simulink model "cybershipII_ctrl_1_nonlin"  (R2020b)
settings: Solver=FixedStepAuto  StartTime=0.0  StopTime=100  FixedStep=0.01  RelTol=1e-3
libraries: simulink x1
settings Model: Creator=ASUS  LastModifiedBy=ASUS

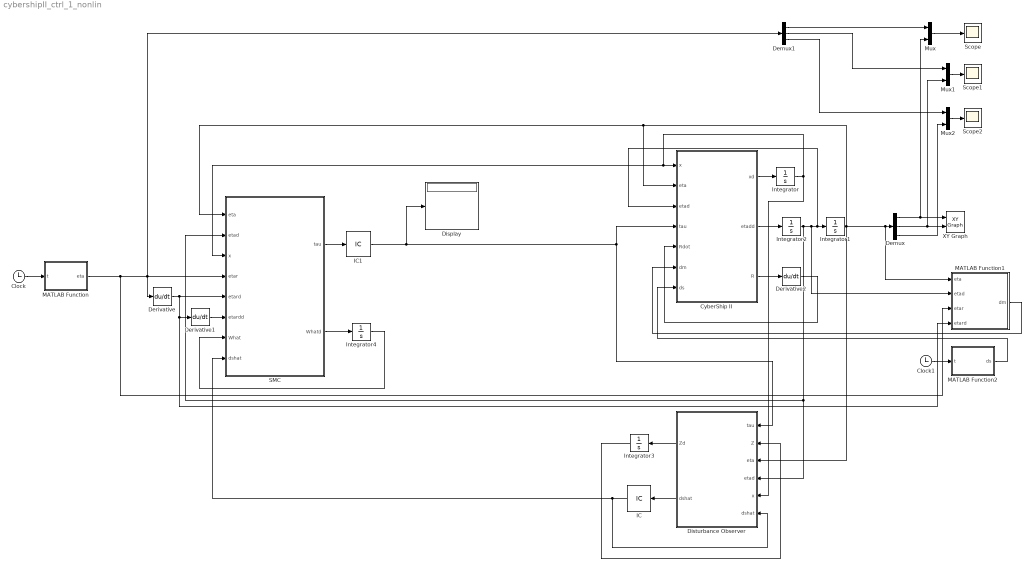
== system cybershipII_ctrl_1_nonlin ==
  Clock : Clock
  Clock1 : Clock
  CyberShip II : MATLAB Function  TreatAsAtomicUnit=on
  Demux : Demux  Outputs=3
  Demux1 : Demux  Outputs=3
  Derivative : Derivative
  Derivative1 : Derivative
  Derivative2 : Derivative
  Display : Display
  Disturbance Observer : MATLAB Function  TreatAsAtomicUnit=on
  IC : InitialCondition  Value=[0; 0; 0]
  IC1 : InitialCondition  Value=[0; 0; 0]
  Integrator : Integrator  InitialCondition=[3; 0; 0]
  Integrator1 : Integrator  InitialCondition=[0; 0; pi/4]
  Integrator2 : Integrator  InitialCondition=[3*cos(pi/4) 3*sin(pi/4) 0]
  Integrator3 : Integrator
  Integrator4 : Integrator
  MATLAB Function : MATLAB Function  TreatAsAtomicUnit=on
  MATLAB Function1 : MATLAB Function  TreatAsAtomicUnit=on
  MATLAB Function2 : MATLAB Function  TreatAsAtomicUnit=on
  Mux : Mux  Inputs=2
  Mux1 : Mux  Inputs=2
  Mux2 : Mux  Inputs=2
  SMC : MATLAB Function  TreatAsAtomicUnit=on
  Scope : Scope
  Scope1 : Scope
  Scope2 : Scope
  XY Graph : simulink/Sinks/XY Graph  xmin=-100  xmax=100  ymin=-100  ymax=100  st=-1
  wires:
  CyberShip II/1(xd) -> Integrator/1
  Integrator1/1 -> SMC/1(eta), CyberShip II/2(eta), MATLAB Function1/1(eta), Demux/1, Disturbance Observer/3(eta)
  Demux/1 -> Mux/2, XY Graph/1
  Demux/2 -> Mux1/2, XY Graph/2
  CyberShip II/3(R) -> Derivative2/1
  Derivative2/1 -> CyberShip II/5(Rdot)
  Integrator/1 -> Disturbance Observer/5(x), SMC/3(x), CyberShip II/1(x)
  CyberShip II/2(etadd) -> Integrator2/1
  Integrator2/1 -> SMC/2(etad), Disturbance Observer/4(etad), MATLAB Function1/2(etad), CyberShip II/3(etad), Integrator1/1
  SMC/1(tau) -> IC1/1
  Disturbance Observer/1(Zd) -> Integrator3/1
  Integrator3/1 -> Disturbance Observer/2(Z)
  IC/1 -> SMC/8(dshat), Disturbance Observer/6("dshat ")
  Disturbance Observer/2(dshat) -> IC/1
  Integrator4/1 -> SMC/7(What)
  Clock/1 -> MATLAB Function/1(t)
  Derivative/1 -> SMC/5(etard), MATLAB Function1/4(etard), Derivative1/1
  SMC/2(Whatd) -> Integrator4/1
  MATLAB Function/1(eta) -> MATLAB Function1/3(etar), SMC/4(etar), Demux1/1, Derivative/1
  Derivative1/1 -> SMC/6(etardd)
  IC1/1 -> Display/1, CyberShip II/4(tau), Disturbance Observer/1(tau)
  Demux1/1 -> Mux/1
  Mux/1 -> Scope/1
  Demux1/2 -> Mux1/1
  Mux1/1 -> Scope1/1
  Demux1/3 -> Mux2/1
  Demux/3 -> Mux2/2
  Mux2/1 -> Scope2/1
  MATLAB Function2/1(ds) -> CyberShip II/7(ds)
  Clock1/1 -> MATLAB Function2/1(t)
  MATLAB Function1/1(dm) -> CyberShip II/6(dm)

== matlab function cybershipII_ctrl_1_nonlin/Disturbance Observer ==
  data: tau input; Zd output; Z input; eta input; etad input; x input; dshat output; dshat input
function [Zd,dshat] = fcn(tau,Z,eta,etad,x,dshat)

u = x(1);
v = x(2);
r = x(3);

m = 23.8;
Izz = 1.76;
XG = 0.046;
Xu = -0.72253;
Yv = -0.88965;
Yr = -7.25;
Nv = 0.0313;
Nr = -1.9;
Xud = -2.0;
Yvd = -10.0;
Yrd = -0.1;
Nvd = 0;
Nrd = -0.1;
xdelr = 1;                      % Longitudinal moment arm from the center of rotation

R = [cos(eta(3)) -sin(eta(3)) 0; sin(eta(3)) cos(eta(3)) 0; 0 0 1];
M0t = [m-Xud 0 0; 0 m-Yvd m*XG-Yrd; 0 m*XG-Nvd Izz-Nrd];
C0t = [0 0 (-M0t(2,2)*v-M0t(2,3)*r); 0 0 M0t(1,1)*u; (M0t(2,2)*v+M0t(2,3)*r) (-M0t(1,1)*u) 0];
D0t = -[Xu 0 0; 0 Yv Yr; 0 Nv Nr];
% M0 = R*M0t*R';
% C0 = R*(C0t-M0t

H = [0.1309 0 0; 0 0.1309 0; 0 0 0.1309];

L = inv(H)*inv(M0t);
P = inv(H)*etad;

% T = del(1);
% del_rudder = del(2);
% tau = [T*cos(del_rudder); -T*sin(del_rudder); xdelr*T*sin(del_rudder)];

Zd = [0; 0; 0];
Zd = L*(C0t*etad + D0t*etad - R*tau) - L*dshat;
dshat = Z + P;

== matlab function cybershipII_ctrl_1_nonlin/CyberShip II ==
  data: x input; eta input; etad input; xd output size=3; tau input; etadd output size=3; R output; Rdot input; dm input; ds input
function [xd,etadd,R] = fcn(x,eta,etad,tau,Rdot,dm,ds)

u = x(1);
v = x(2);
r = x(3);
% T = del(1);
% del_rudder = del(2);

m = 23.8;
Izz = 1.76;
XG = 0.046;
Xu = -0.72253;
Yv = -0.88965;
Yr = -7.25;
Nv = 0.0313;
Nr = -1.9;
Xud = -2.0;
Yvd = -10.0;
Yrd = -0.1;
Nvd = 0;
Nrd = -0.1;
xdelr = 1;                      % Longitudinal moment arm from the center of rotation

M0t = [m-Xud 0 0; 0 m-Yvd m*XG-Yrd; 0 m*XG-Nvd Izz-Nrd];
C0t = [0 0 -M0t(2,2)*v-M0t(2,3)*r; 0 0 M0t(1,1)*u; M0t(2,2)*v+M0t(2,3)*r -M0t(1,1)*u 0];
D0t = -[Xu 0 0; 0 Yv Yr; 0 Nv Nr];

xd = [0; 0; 0];
xd = inv(M0t)*(tau - C0t*x - D0t*x);

R = [cos(eta(3)) -sin(eta(3)) 0; sin(eta(3)) cos(eta(3)) 0; 0 0 1];

M0 = R*M0t*R';
C0 = R*(C0t-M0t*R'*Rdot)*R';
D0 = R*D0t*R';

etadd = inv(M0)*(R*tau + dm + ds - C0*etad - D0*etad);

% delta = [0; 0; 0; 0];
% 
% V = [x(1); x(2); x(4)];
% R = [cos(x(3)) -sin(x(3)) 0; sin(x(3)) cos(x(3)) 0; 0 0 1];
% etad = R*V;

== matlab function cybershipII_ctrl_1_nonlin/SMC ==
  data: eta input; etad input; x input; tau output; etar input; etard input; etardd input; What input; dshat input; Whatd output
function [tau,Whatd] = fcn(eta,etad,x,etar,etard,etardd,What,dshat)

e = eta - etar;
ed = etad - etard;
K = [10 0 0; 0 10 0; 0 0 10];
s = K*e + ed;
delta = 0.1;

sat = [0; 0; 0];

for i = 1:3
    if abs(s(i)) > delta
        sat(i) = sign(s(i));
    else
        sat(i) = (1/delta)*s(i)*abs(s(i));
    end
end

R = [cos(eta(3)) -sin(eta(3)) 0; sin(eta(3)) cos(eta(3)) 0; 0 0 1];    

u = x(1);
v = x(2);
r = x(3);

m = 23.8;
Izz = 1.76;
XG = 0.046;
Xu = -0.72253;
Yv = -0.88965;
Yr = -7.25;
Nv = 0.0313;
Nr = -1.9;
Xud = -2.0;
Yvd = -10.0;
Yrd = -0.1;
Nvd = 0;
Nrd = -0.1;
xdelr = 1;                      % Longitudinal moment arm from the center of rotation

M0t = [m-Xud 0 0; 0 m-Yvd m*XG-Yrd; 0 m*XG-Nvd Izz-Nrd];
C0t = [0 0 (-M0t(2,2)*v-M0t(2,3)*r); 0 0 M0t(1,1)*u; (M0t(2,2)*v+M0t(2,3)*r) (-M0t(1,1)*u) 0];
D0t = -[Xu 0 0; 0 Yv Yr; 0 Nv Nr];

rho = -M0t*(etardd-K*ed)-C0t*(etard-K*e)-D0t*etad;
Kv = [100 0 0; 0 100 0; 0 0 100];
xi = [100 0 0; 0 100 0; 0 0 100];


p = [etard(1) ed(1) etar(1) e(1); 
    etard(2) ed(2) etar(2) e(2); 
    etard(3) ed(3) etar(3) e(3)];

c_upper = [2 2 2 2; 2 2 2 2; 0.5 0.5 0.5 0.5];
c_step = [1 1 1 1; 1 1 1 1; 0.25 0.25 0.25 0.25];

neural_num = 5;
c = zeros(3,4,neural_num);
c(:,:,1) = c_upper;
bj = 10;

h = zeros(3, neural_num);
for i = 1:neural_num
   h(1,i) = exp(-norm(p(1,:)-c(1,:,i))^2/(bj^2));
   h(2,i) = exp(-norm(p(2,:)-c(2,:,i))^2/(bj^2));
   h(2,i) = exp(-norm(p(3,:)-c(3,:,i))^2/(bj^2));
   c(:,:,i) = c(:,:,i) - c_step;
end
learn_rate = 0.1;

Whatd = zeros(3, neural_num);
for i = 1:3
    Whatd(i,:) = ((1/learn_rate)*s(i)).*h(i,:);
end

and = [0.5; 0.5; 0.1];
dmhat = zeros(3,1);
for i = 1:3
    for j = 1:neural_num
        dmhat(i) = dmhat(i)+What(i,j)*h(i,j);
    end   
    dmhat(i) = dmhat(i) + and(i);
end

tau = -R'*(rho+Kv*s+xi*sat+dshat);

== matlab function cybershipII_ctrl_1_nonlin/MATLAB Function1 ==
  data: dm output; eta input; etad input; etar input; etard input
function dm = fcn(eta, etad, etar,etard)

xr = etar(1);
yr = etar(2);
psir = etar(3);

xrd = etard(1);
yrd = etard(2);
psird = etard(3);

x = eta(1);
y = eta(2);
psi = eta(3);

xd = etad(1);
yd = etad(2);
psid = etad(3);

dmx = 2*cos(xrd)+sin(xr)+2*sin(x-xr)+2*cos(xd-xrd);
dmy = 3*cos(yrd)+sin(yr)+4*sin(y-yr)+2.5*cos(yd-yrd);
dmpsi = 0.4*cos(psird)+0.3*sin(psir)+4*sin(psi-psir)+2*cos(psid - psird);

dm = [dmx; dmy; dmpsi];

== matlab function cybershipII_ctrl_1_nonlin/MATLAB Function ==
  data: t input; eta output
function eta = fcn(t)
%#codegen

eta = [10;15;0];

== matlab function cybershipII_ctrl_1_nonlin/MATLAB Function2 ==
  data: ds output; t input
function ds = fcn(t)

dsx = 15 + 0.2*sin(0.1*pi*t-pi/3)+0.3*cos(0.3*pi*t+pi/4);
dsy = 17 + 0.3*sin(0.2*pi*t+pi/4)+0.4*cos(0.1*pi*t-pi/6);
dspsi = 7 + 0.5*sin(0.3*pi*t+pi/6)+0.15*cos(0.2*pi*t-pi/3);

ds = [dsx; dsy; dspsi];
